simulink model "Adaptive_Equalyzer_1"  (Simulink 7.7)
settings: Solver=VariableStepDiscrete  StartTime=0.0  StopTime=60  RelTol=1e-3
undefined symbols (not defined in the file or in its folder): magnitude
libraries: simulink x3, dspsnks4 x3, dspadpt3 x1
settings Model: Creator=horacio  LastModifiedBy=horacio

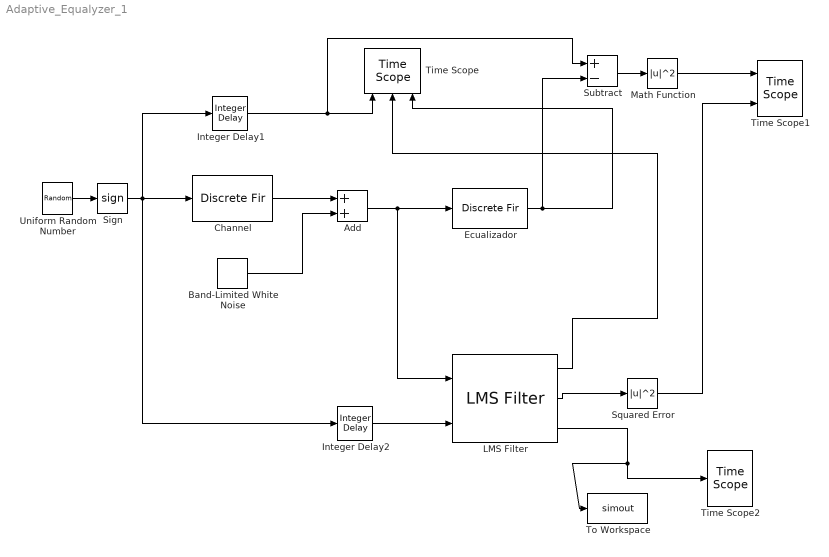
== system Adaptive_Equalyzer_1 ==
  Add : Sum
  Band-Limited White Noise : simulink/Sources/Band-Limited White Noise  SystemSampleTime=-1  Cov=[1e-6]  Ts=0.1  seed=[23341]
  Channel : DiscreteFir  NumCoeffs=actual_isi
  Ecualizador : DiscreteFir  NumCoeffs=coeficientes
  Integer Delay1 : simulink/Discrete/Integer Delay  NumDelays=10  vinit=0.0  samptime=-1
  Integer Delay2 : simulink/Discrete/Integer Delay  NumDelays=10  vinit=0.0  samptime=-1
  LMS Filter : dspadpt3/LMS Filter  Algo=LMS  L=11  stepflag=Dialog  mu=0.115  leakage=1.0  ic=0  Adapt=off  resetflag=None  weights=on  secondCoeffMode=User-defined  secondCoeffWordLength=2  secondCoeffFracLength=15  accum2Mode=User-defined  accum2FracLength=20  prodOutput2Mode=User-defined  prodOutput2FracLength=20  prodOutput3Mode=User-defined  prodOutput3FracLength=20  prodOutput4Mode=User-defined  prodOutput4FracLength=20  quotientMode=User-defined  quotientFracLength=20  roundingMode=Floor  overflowMode=off  addnparflag=off
  Math Function : Math  Operator=magnitude^2  SaturateOnIntegerOverflow=on
  Sign : Signum
  Squared Error : Math  Operator=magnitude^2  SaturateOnIntegerOverflow=on
  Subtract : Sum  Inputs=+-
  Time Scope : dspsnks4/Time Scope  NumInputPorts=3
  Time Scope1 : dspsnks4/Time Scope  NumInputPorts=2
  Time Scope2 : dspsnks4/Time Scope
  To Workspace : ToWorkspace  VariableName=simout  SampleTime=-1  SaveFormat=Structure With Time
  Uniform Random Number : UniformRandomNumber  Seed=1  SampleTime=0.1
  wires:
  Sign/1 -> Channel/1, Integer Delay1/1, Integer Delay2/1
  Uniform Random Number/1 -> Sign/1
  Integer Delay1/1 -> Time Scope/1, Subtract/1
  Ecualizador/1 -> Subtract/2, Time Scope/3
  Channel/1 -> Add/1
  Band-Limited White Noise/1 -> Add/2
  Add/1 -> Ecualizador/1, LMS Filter/1
  Subtract/1 -> Math Function/1
  Math Function/1 -> Time Scope1/1
  Integer Delay2/1 -> LMS Filter/2
  LMS Filter/2 -> Squared Error/1
  Squared Error/1 -> Time Scope1/2
  LMS Filter/1 -> Time Scope/2
  LMS Filter/3 -> Time Scope2/1, To Workspace/1
